simulink model "ackermann"  (R2023b)
settings: Solver=ode4  StartTime=0.0  StopTime=200  FixedStep=0.001  RelTol=1e-3
settings Model: Creator=Admin  LastModifiedBy=Admin

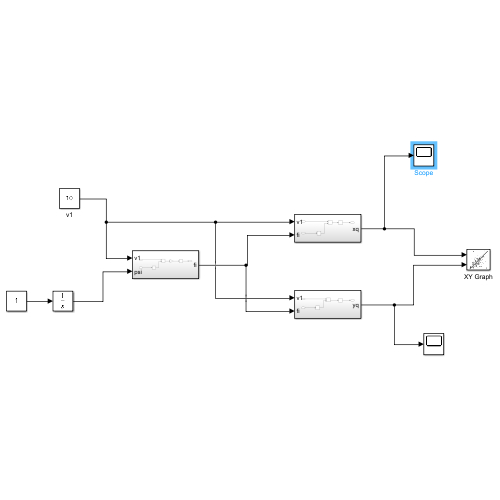
[thumbnail: Simulink's stored preview of the top-level diagram]
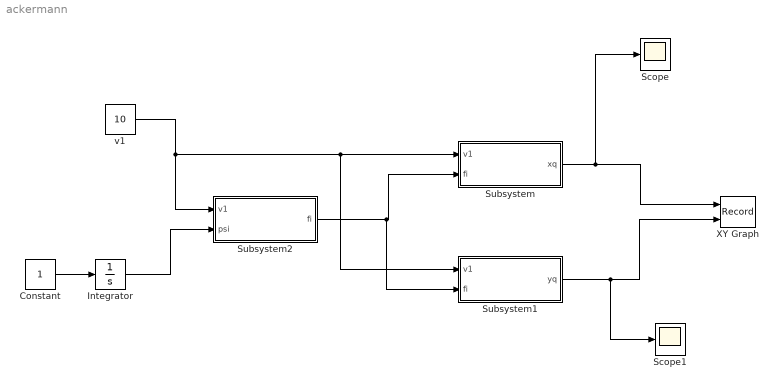
== system ackermann ==
  Constant : Constant
  Integrator : Integrator
  Scope : Scope
  Scope1 : Scope
  Subsystem : Subsystem
  Subsystem1 : Subsystem
  Subsystem2 : Subsystem
  XY Graph : Record  FileSettingsInternal="{\"entries\":[{\"content\":{\"excelSettings\":{\"content\":{},\"type\":\"Streamout.ExcelSettings\"}},\"type\":\"Streamout.FileSettingStorage\",\"uuid\":\"\"}],\"packageUris\":[\"http:\\/\\/schema.mathworks.com\\/mf0\\/streamout_blocks\\/R2020a\"],\"version\":\"1.0\"}"  Layout=[1 1]  SignalsInternal="{\"entries\":[{\"content\":{\"signals\":[{\"content\":{\"blockPath\":[],\"dimensions\":[1],\"domain\":\"\",\"lineColor\":\"#fe330a\",\"port\":1,\"sid\":[\"\"],\"signalID\":144,\"signalName\":\"Subsystem\"},\"type\":\"RecordBlkView.Signal\",\"uuid\":\"\"},{\"content\":{\"blockPath\":[],\"dimensions\":[1],\"domain\":\"\",\"lineColor\":\"#22b573\",\"port\":2,\"sid\":[\"\"],\"signalID\":148,\"signalName\":\"Subsystem1\"},\"type\":\"RecordBlkView.Signal\",\"uuid\":\"\"}]},\"type\":\"RecordBlkView.InputSignals\",\"uuid\":\"\"}],\"packageUris\":[\"http:\\/\\/schema.mathworks.com\\/mf0\\/streamout_blocks\\/R2020a\"],\"version\":\"1.0\"}"  VisualizationBindings="{\"xyplotplugin\":{\"info\":[{\"series\":[],\"subplotID\":1}]}}"  CompatibilityTag=XY
  v1 : Constant  Value=10
  wires:
  Subsystem2/1(fi) -> Subsystem1/2(fi), Subsystem/2(fi)
  Subsystem/1(xq) -> Scope/1, XY Graph/1
  Subsystem1/1(yq) -> Scope1/1, XY Graph/2
  v1/1 -> Subsystem1/1(v1), Subsystem/1(v1), Subsystem2/1(v1)
  Constant/1 -> Integrator/1
  Integrator/1 -> Subsystem2/2(psi)

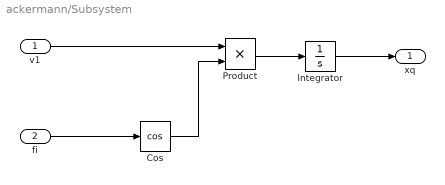
== system ackermann/Subsystem ==
  v1 : Inport
  fi : Inport  Port=2
  Cos : Trigonometry  Operator=cos
  Integrator : Integrator
  Product : Product
  xq : Outport
  wires:
  fi/1 -> Cos/1
  v1/1 -> Product/1
  Cos/1 -> Product/2
  Product/1 -> Integrator/1
  Integrator/1 -> xq/1

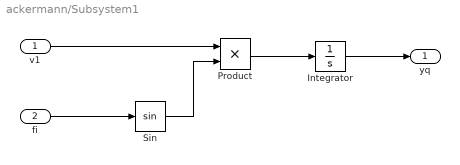
== system ackermann/Subsystem1 ==
  v1 : Inport
  fi : Inport  Port=2
  Integrator : Integrator
  Product : Product
  Sin : Trigonometry
  yq : Outport
  wires:
  fi/1 -> Sin/1
  v1/1 -> Product/1
  Sin/1 -> Product/2
  Product/1 -> Integrator/1
  Integrator/1 -> yq/1

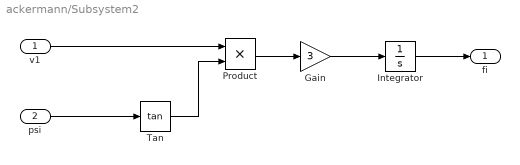
== system ackermann/Subsystem2 ==
  v1 : Inport
  psi : Inport  Port=2
  Gain : Gain  Gain=3
  Integrator : Integrator
  Product : Product
  Tan : Trigonometry  Operator=tan
  fi : Outport
  wires:
  psi/1 -> Tan/1
  v1/1 -> Product/1
  Tan/1 -> Product/2
  Product/1 -> Gain/1
  Gain/1 -> Integrator/1
  Integrator/1 -> fi/1
